simulink model "sl_subsys_fcncall4"  (Simulink 7.6)
settings: Solver=FixedStepDiscrete  StartTime=0.0  StopTime=10.0  FixedStep=1  RelTol=1e-3
Description:
  | Enabled subsystem containing function-call initiator with data sharing
  | 
  | The enabled subsystem below contains a Stateflow chart invoking the functions f() and g().
  | Referring back to the demo model sl_subsys_fcncall3.mdl, you'll find that the enabled
  | subsystem is a common function-call initiator of both f() and g(), thus the signal,
  | d2 is treated as a data store.
settings Model: Creator=The MathWorks Inc.  CovMetricSettings=d  ExtModeAutoUpdateStatusClock=off
settings OptimizationCC: BlockReduction=off  BooleanDataType=off  InlineInvariantSignals=on  InitFltsAndDblsToZero=on
settings DebuggingCC: SaveWithParameterizedLinksMsg=none  SignalResolutionControl=TryResolveAllWithWarning  SolverPrmCheckMsg=none  MultiTaskDSMMsg=warning  MultiTaskCondExecSysMsg=none
settings HardwareCC: TargetUnknown=on
settings SFSimCC: SimParseCustomCode=off
settings RTWCC: IncludeERTFirstTime=on
settings CodeAppCC: CustomSymbolStrFcn=$F$N$M
settings GRTTargetCC: TargetFcnLib=ansi_tfl_tmw.mat

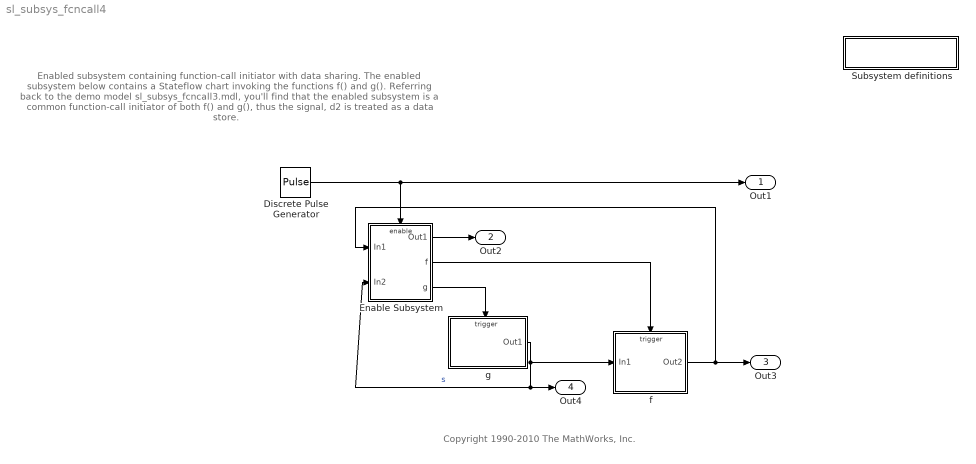
== system sl_subsys_fcncall4 ==
  note: Enabled subsystem containing function-call initiator with data sharing.
      |
      | The enabled subsystem below contains a Stateflow chart invoking the functions f() and g().
      | Referring back to the demo model sl_subsys_fcncall3.mdl, you'll find that the enabled
      | subsystem is a common function-call initiator of both f() and g(), thus the signal,
      | d2 is treated as a data store.
  note: Copyright 1990-2010 The MathWorks, Inc.
  " Subsystem definitions" : Subsystem
      settings: OpenFcn=helpview([matlabroot,'/toolbox/simulink/simdemos/simfeatures/html/sl_subsys_definitions.html']);
      mask Display: disp('Subsystem\ndefinitions')
  Discrete Pulse Generator : DiscretePulseGenerator
  Enable Subsystem : Subsystem  TreatAsAtomicUnit=on
  f : Subsystem  TreatAsAtomicUnit=on
  g : Subsystem  TreatAsAtomicUnit=on
  Out1 : Outport
  Out2 : Outport  Port=2
  Out3 : Outport  Port=3
  Out4 : Outport  Port=4
  wires:
  Enable Subsystem/3(g) -> g/Trigger
  g/1(Out1) -> f/1(In1), Enable Subsystem/2(In2), Out4/1  "s"
  f/1(Out2) -> Enable Subsystem/1(In1), Out3/1
  Enable Subsystem/1(Out1) -> Out2/1
  Enable Subsystem/2(f) -> f/Trigger
  Discrete Pulse Generator/1 -> Enable Subsystem/Enable, Out1/1

== system sl_subsys_fcncall4/ Subsystem definitions ==

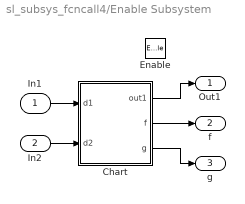
== system sl_subsys_fcncall4/Enable Subsystem ==
  In1 : Inport
  In2 : Inport  Port=2
  Enable : EnablePort
  Chart : Stateflow chart  TreatAsAtomicUnit=on
  Out1 : Outport
  f : Outport  Port=2
  g : Outport  Port=3
  wires:
  In1/1 -> Chart/1(d1)
  In2/1 -> Chart/2(d2)
  Chart/1(out1) -> Out1/1
  Chart/2(f) -> f/1
  Chart/3(g) -> g/1

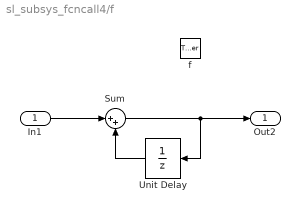
== system sl_subsys_fcncall4/f ==
  In1 : Inport
  f : TriggerPort  TriggerType=function-call
  Sum : Sum  Inputs=|++  SaturateOnIntegerOverflow=on  InputSameDT=on  OutDataTypeStr=Inherit: Same as first input
  Unit Delay : UnitDelay  SampleTime=-1
  Out2 : Outport
  wires:
  In1/1 -> Sum/1
  Unit Delay/1 -> Sum/2
  Sum/1 -> Out2/1, Unit Delay/1

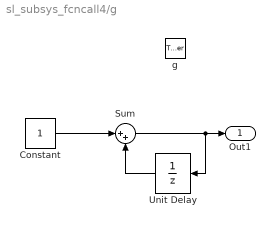
== system sl_subsys_fcncall4/g ==
  g : TriggerPort  TriggerType=function-call
  Constant : Constant
  Sum : Sum  Inputs=|++  SaturateOnIntegerOverflow=on  InputSameDT=on  OutDataTypeStr=Inherit: Same as first input
  Unit Delay : UnitDelay  SampleTime=-1
  Out1 : Outport
  wires:
  Constant/1 -> Sum/1
  Unit Delay/1 -> Sum/2
  Sum/1 -> Out1/1, Unit Delay/1

== stateflow chart Enable Subsystem/Chart ==
  state one/
    entry: f; out1= d1+d2;
  state two/
    entry: g; out1=d1-d2;
  one -> two
  two -> one
  (default) -> one
  data: d1 input double; d2 input double; out1 output double
  events: f output FUNCTION_CALL_EVENT; g output FUNCTION_CALL_EVENT
